simulink model "pospoli_XY_traiettoria_discretizzato"  (R2020b)
settings: Solver=VariableStepAuto  StartTime=0.0  StopTime=3  RelTol=1e-3
values from neighbouring files (symbols this model uses):
  Acc_asse_x = []    [main_Strategia_di_pilotaggio.m]
  Acc_asse_y = []    [main_Strategia_di_pilotaggio.m]
  Gppx_agg_rc = 0.4    [main_Strategia_di_pilotaggio.m]
  Gppx_agg_rm = 1    [main_Strategia_di_pilotaggio.m]
  Gppy_agg_rc = 0.8    [main_Strategia_di_pilotaggio.m]
  Gppy_agg_rm = 1    [main_Strategia_di_pilotaggio.m]
  mx = config_dc_x(parx)    [Main_traiettoria.m]    (also in Main_traiettoria_ordinato.m; main_Strategia_di_pilotaggio.m)
  my = config_dc_y(pary)    [Main_traiettoria.m]    (also in Main_traiettoria_ordinato.m; main_Strategia_di_pilotaggio.m)
  ppx_c = pos_poli_cc_x(mx, acx, 2)    [main_Strategia_di_pilotaggio.m]
  ppx_m = pos_poli_cc_x(mx, acx, 1)    [main_Strategia_di_pilotaggio.m]
  ppy_c = pos_poli_cc_y(my, acy, 2)    [main_Strategia_di_pilotaggio.m]
  ppy_m = pos_poli_cc_y(my, acy, 1)    [main_Strategia_di_pilotaggio.m]
  time = 0:tf/np:tf    [Main_traiettoria.m]    (also in Main_traiettoria_ordinato.m = 0:passo:tsim)
  Vel_asse_x = []    [main_Strategia_di_pilotaggio.m]
  Vel_asse_y = []    [main_Strategia_di_pilotaggio.m]
  x = zeros(length(time),1)    [Main_traiettoria.m]    (also in Main_traiettoria_ordinato.m; main_Strategia_di_pilotaggio.m = [])
  y = zeros(length(time),1)    [Main_traiettoria.m]    (also in Main_traiettoria_ordinato.m; main_Strategia_di_pilotaggio.m = [])
undefined symbols (not defined in the file or in its folder): accelerazioni, accelerazioniy, ci_x, ci_y, interpolazione_tempi, parx, pary
libraries: simulink x6
settings Model: Creator=stefa  LastModifiedBy=user
settings DebuggingCC: SFMachineParentedDataDiag=error

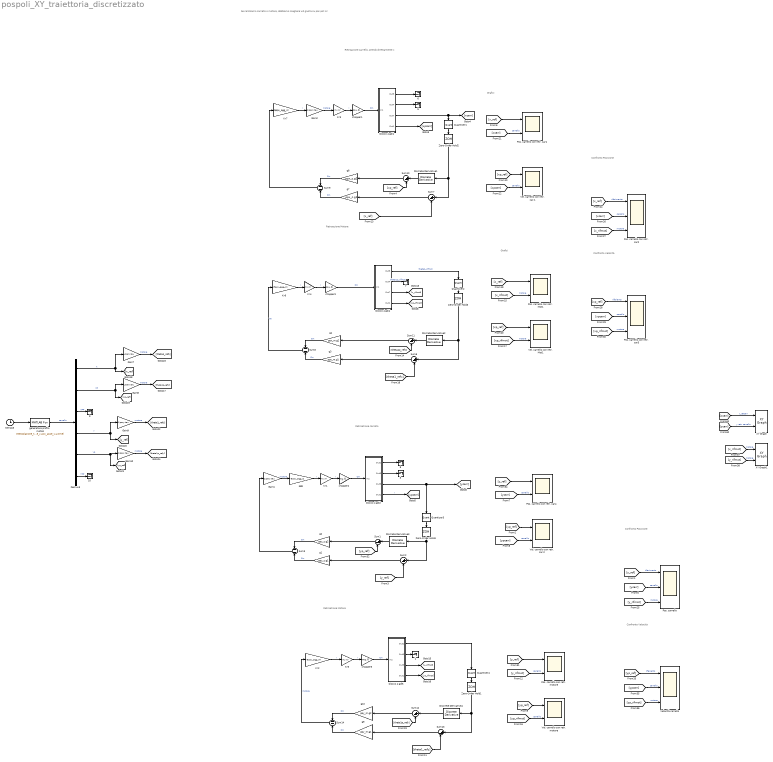
== system pospoli_XY_traiettoria_discretizzato ==
  note: Confronto Posizione
  note: Confronto
      | Velocità
  note: Retroazione Motore
  note: Grafici
  note: Grafici
  note: Retroazione carrello, prendo direttamente x
  note: Retroazione carrello
  note: Confronto
      | Velocità
  note: Retroazione Motore
  note: Confronto Posizione
  note: Se cambiamo carrello o motore, dobbiamo scegliere w0 giusta su pos poli cc
   {1,3,5..10} (8 alike) : Terminator
  Demux3 : Demux  Outputs=6
  Discrete Derivative1 : simulink/Discrete/Discrete Derivative  gainval=1  ICPrevScaledInput=0.0  OutMin=[]  OutMax=[]  OutDataType=fixdt(1, 16)  OutScaling=2^-10  DoSatur=off
  Discrete Derivative2 : simulink/Discrete/Discrete Derivative  gainval=1.0  ICPrevScaledInput=0.0  OutMin=[]  OutMax=[]  OutDataType=fixdt(1, 16)  OutScaling=2^-10  DoSatur=off
  Discrete Derivative3 : simulink/Discrete/Discrete Derivative  gainval=1  ICPrevScaledInput=0.0  OutMin=[]  OutMax=[]  OutDataType=fixdt(1, 16)  OutScaling=2^-10  DoSatur=off
  Discrete Derivative4 : simulink/Discrete/Discrete Derivative  gainval=1.0  ICPrevScaledInput=0.0  OutMin=[]  OutMax=[]  OutDataType=fixdt(1, 16)  OutScaling=2^-10  DoSatur=off
  Gain1 : Gain  Gain=1/pary.tau
  Gain10 : Gain  Gain=1/pary.tau
  Gain2 : Gain  Gain=1/parx.tau
  Gain7 : Gain  Gain=1/parx.tau
  Gain8 : Gain  Gain=1/parx.tau
  Gain9 : Gain  Gain=1/pary.tau
  Kr1 : Gain  Gain=my.Kr
  Kr2 : Gain  Gain=Gppy_agg_rm
  Kr3 : Gain  Gain=mx.Kr
  Kr4 : Gain  Gain=mx.Kr
  Kr5 : Gain  Gain=my.Kr
  Kr6 : Gain  Gain=Gppx_agg_rm
  Kr7 : Gain  Gain=Gppx_agg_rc
  "Pos. carrello " : Scope  NumInputPorts=3
  Pos. carrello con retr. Mot1 : Scope  NumInputPorts=2
  Pos. carrello con retr. car1 : Scope  NumInputPorts=2
  Pos. carrello con retr. car2 : Scope  NumInputPorts=3
  Pos. carrello con retr. car3 : Scope  NumInputPorts=3
  Pos. carrello con retr. car4 : Scope  NumInputPorts=2
  Pos. carrello con retr. motore : Scope  NumInputPorts=2
  Quantizer{1..4} (4 alike) : Quantizer  QuantizationInterval=10/4096
  Sum{1..2,6..7,10..13} (8 alike) : Sum  Inputs=|+-
  Sum{3,8..9,14} (4 alike) : Sum  Inputs=--
  Vel. carrello con retr. Mot1 : Scope  NumInputPorts=2
  Vel. carrello con retr. car.1 : Scope  NumInputPorts=2
  Vel. carrello con retr. car.2 : Scope  NumInputPorts=2
  Vel. carrello con retr. motore : Scope  NumInputPorts=2
  Velocità carrello : Scope  NumInputPorts=3
  XY Graph : simulink/Sinks/XY Graph  xmin=-0.5  xmax=0.5  ymin=-0.5  ymax=0.5  st=-1
  XY Graph1 : simulink/Sinks/XY Graph  xmin=-0.5  xmax=0.5  ymin=-0.5  ymax=0.5  st=-1
  Zero-Order Hold{1..4} (4 alike) : ZeroOrderHold  SampleTime=0.001
  agg : Gain  Gain=Gppy_agg_rc
  blocco 4 gdl1 : Subsystem
  blocco 4 gdl2 : Subsystem
  blocco 4 gdl4 : Subsystem
  blocco 4 gdl5 : Subsystem
  chopper1 : Gain  Gain=mx.K
  chopper2 : Gain  Gain=my.K
  chopper3 : Gain  Gain=mx.K
  chopper5 : Gain  Gain=my.K
  g1 : Gain  Gain=ppy_c.g1
  g10 : Gain  Gain=ppy_m.g2
  g2 : Gain  Gain=ppy_c.g2
  g3 : Gain  Gain=ppx_m.g1
  g4 : Gain  Gain=ppx_m.g2
  g7 : Gain  Gain=ppx_c.g1
  g8 : Gain  Gain=ppx_c.g2
  g9 : Gain  Gain=ppy_m.g1
  generatore profilo moto3 : MATLABFcn  MATLABFcn=interpolazione_tempi(x,Vel_asse_x,Acc_asse_x,y,Vel_asse_y,Acc_asse_y,u,time)  OutputDimensions=6
  tempo3 : Clock
      settings: Decimation=tsim
  wires:
  blocco 4 gdl4/2(Out4) -> " 7"/1  "theta1p_rifmot"
  chopper3/1 -> blocco 4 gdl4/1(In1)  "Cm"
  Discrete Derivative2/1 -> Sum11/1
  Quantizer2/1 -> Zero-Order Hold3/1
  [xcarr] -> Pos. carrello con retr. car2/2  "carrello"
  [xp_rifmot] -> Pos. carrello con retr. car3/3  "motore"
  blocco 4 gdl4/1(Out3) -> Quantizer2/1  "theta1_rifmot"
  [theta1_refx] -> Sum6/2
  [xp_rifmot] -> Vel. carrello con retr. Mot1/2  "motore"
  [xp_ref] -> Vel. carrello con retr. car.1/1
  g4/1 -> Sum8/1  "Cm"
  Kr4/1 -> chopper3/1  "I"
  blocco 4 gdl1/3(Out7) -> Quantizer1/1, [xcarr]
  blocco 4 gdl1/4(Out1) -> [xpcarr]
  blocco 4 gdl4/4(Out1) -> [xp_rifmot]
  [xp_ref] -> Sum10/2
  blocco 4 gdl4/3(Out7) -> [x_rifmot]
  g7/1 -> Sum9/2  "Cm"
  chopper1/1 -> blocco 4 gdl1/1(In1)  "Cm"
  [x_rifmot] -> Pos. carrello con retr. Mot1/2  "motore"
  g8/1 -> Sum9/1  "Cm"
  blocco 4 gdl1/1(Out3) -> " 6"/1
  [x_ref] -> Sum7/2
  [xpcarr] -> Pos. carrello con retr. car3/2  "carrello"
  Sum11/1 -> g4/1
  [x_ref] -> Pos. carrello con retr. car2/1  "riferimento"
  [xp_ref] -> Vel. carrello con retr. Mot1/1
  blocco 4 gdl1/2(Out4) -> " 5"/1
  [x_ref] -> Pos. carrello con retr. Mot1/1
  [xp_ref] -> Pos. carrello con retr. car3/1  "riferiento"
  [xpcarr] -> Vel. carrello con retr. car.1/2  "carrello"
  Quantizer1/1 -> Zero-Order Hold2/1
  Sum6/1 -> g3/1
  [xcarr] -> Pos. carrello con retr. car1/2  "carrello"
  Discrete Derivative1/1 -> Sum10/1
  [x_rifmot] -> Pos. carrello con retr. car2/3  "motore"
  [theta1p_refx] -> Sum11/2
  g3/1 -> Sum8/2  "Cm"
  Sum10/1 -> g8/1
  [x_ref] -> Pos. carrello con retr. car1/1
  Sum7/1 -> g7/1
  Kr3/1 -> chopper1/1  "I"
  [y_ref] -> Pos. carrello con retr. motore/1
  Sum12/1 -> g10/1
  blocco 4 gdl5/4(Out1) -> [yp_rifmot]
  blocco 4 gdl5/3(Out3) -> [y_rifmot]
  g2/1 -> Sum3/1  "Cm"
  chopper5/1 -> blocco 4 gdl5/1(In2)  "Cm"
  [ycarr] -> Pos. carrello con retr. car4/2  "carrello"
  blocco 4 gdl2/3(Out3) -> [ycarr], Quantizer3/1
  [yp_ref] -> Vel. carrello con retr. car.2/1
  Sum2/1 -> g1/1
  blocco 4 gdl2/4(Out1) -> [ypcarr]  "I"
  blocco 4 gdl5/2(Out5) -> " 1"/1
  [ypcarr] -> Velocità carrello/2  "carrello"
  chopper2/1 -> blocco 4 gdl2/1(In2)  "Cm"
  [y_ref] -> Pos. carrello con retr. car4/1
  Kr5/1 -> chopper5/1  "I"
  Sum13/1 -> g9/1
  [yp_ref] -> Vel. carrello con retr. motore/1
  Sum3/1 -> Gain1/1
  [theta1_refy] -> Sum13/2
  [y_ref] -> Sum2/2
  [ycarr] -> "Pos. carrello "/2  "carrello"
  Discrete Derivative4/1 -> Sum12/1
  g1/1 -> Sum3/2  "Cm"
  [y_rifmot] -> Pos. carrello con retr. motore/2  "carrello"
  g9/1 -> Sum14/2  "Cm"
  blocco 4 gdl2/1(Out2) -> " 8"/1
  Quantizer4/1 -> Zero-Order Hold1/1
  blocco 4 gdl2/2(Out5) -> " 3"/1
  [yp_rifmot] -> Velocità carrello/3  "motore"
  [theta1p_refy] -> Sum12/2
  [yp_ref] -> Velocità carrello/1  "riferiento"
  [yp_ref] -> Sum1/2
  blocco 4 gdl5/1(Out2) -> Quantizer4/1
  Sum1/1 -> g2/1
  [y_rifmot] -> "Pos. carrello "/3  "motore"
  Zero-Order Hold4/1 -> Discrete Derivative3/1, Sum2/1
  [yp_rifmot] -> Vel. carrello con retr. motore/2  "carrello"
  Zero-Order Hold1/1 -> Sum13/1, Discrete Derivative4/1
  Quantizer3/1 -> Zero-Order Hold4/1
  Discrete Derivative3/1 -> Sum1/1
  [y_ref] -> "Pos. carrello "/1  "riferimento"
  Kr1/1 -> chopper2/1  "I"
  [ypcarr] -> Vel. carrello con retr. car.2/2  "carrello"
  g10/1 -> Sum14/1  "Cm"
  Demux3/2 -> Gain8/1, [xp_ref]  "XP"
  Gain10/1 -> [theta1p_refy]  "motore"
  Demux3/4 -> [y_ref], Gain9/1  "Y"
  Demux3/1 -> [x_ref], Gain7/1  "X"
  Gain8/1 -> [theta1p_refx]  "motore"
  tempo3/1 -> generatore profilo moto3/1
  Demux3/6 -> " 10"/1  "YPP"
  Demux3/3 -> " 9"/1  "XPP"
  generatore profilo moto3/1 -> Demux3/1  "carrello"
  Demux3/5 -> [yp_ref], Gain10/1  "YP"
  Gain7/1 -> [theta1_refx]  "motore"
  Gain9/1 -> [theta1_refy]  "motore"
  [ycarr] -> XY Graph/2  "y retr. carrello"
  [xcarr] -> XY Graph/1  "x_retcarr"
  Zero-Order Hold2/1 -> Sum7/1, Discrete Derivative1/1
  Zero-Order Hold3/1 -> Discrete Derivative2/1, Sum6/1
  Gain2/1 -> Kr3/1  "motore"
  Gain1/1 -> agg/1  "motore"
  agg/1 -> Kr1/1  "I"
  [x_rifmot] -> XY Graph1/1  "motore"
  [y_rifmot] -> XY Graph1/2  "motore"
  Kr2/1 -> Kr5/1  "I"
  Sum14/1 -> Kr2/1  "motore"
  Kr6/1 -> Kr4/1  "I"
  Sum8/1 -> Kr6/1  "Va"
  Kr7/1 -> Gain2/1  "I"
  Sum9/1 -> Kr7/1

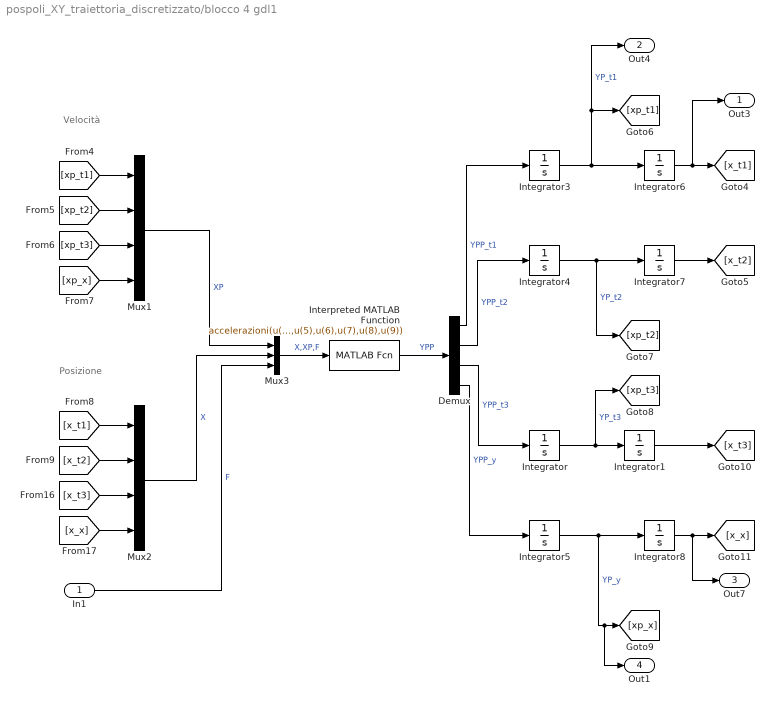
== system pospoli_XY_traiettoria_discretizzato/blocco 4 gdl1 ==
  note: Posizione
  note: Velocità
  In1 : Inport
  Demux : Demux
  Integrator{,3..5} (4 alike) : Integrator
  Integrator1 : Integrator  InitialCondition=ci_x(3)
  Integrator6 : Integrator  InitialCondition=ci_x(1)
  Integrator7 : Integrator  InitialCondition=ci_x(2)
  Integrator8 : Integrator  InitialCondition=ci_x(4)
  Interpreted MATLAB Function : MATLABFcn  MATLABFcn=accelerazioni(u(1),u(2),u(3),u(4),u(5),u(6),u(7),u(8),u(9))  OutputDimensions=4
  Mux1 : Mux
  Mux2 : Mux
  Mux3 : Mux  Inputs=3
  Out3 : Outport
  Out4 : Outport  Port=2
  Out7 : Outport  Port=3
  Out1 : Outport  Port=4
  wires:
  [xp_t3] -> Mux1/3
  Interpreted MATLAB Function/1 -> Demux/1  "YPP"
  Integrator3/1 -> Out4/1, [xp_t1], Integrator6/1  "YP_t1"
  Integrator8/1 -> Out7/1, [x_x]
  Integrator7/1 -> [x_t2]
  [xp_x] -> Mux1/4
  [x_t1] -> Mux2/1
  Mux1/1 -> Mux3/1  "XP"
  [x_x] -> Mux2/4
  Demux/3 -> Integrator/1  "YPP_t3"
  Integrator/1 -> Integrator1/1, [xp_t3]  "YP_t3"
  Mux2/1 -> Mux3/2  "X"
  Integrator6/1 -> Out3/1, [x_t1]
  Integrator5/1 -> Out1/1, [xp_x], Integrator8/1  "YP_y"
  [xp_t2] -> Mux1/2
  Mux3/1 -> Interpreted MATLAB Function/1  "X,XP,F"
  [x_t3] -> Mux2/3
  In1/1 -> Mux3/3  "F"
  Demux/4 -> Integrator5/1  "YPP_y"
  Integrator4/1 -> [xp_t2], Integrator7/1  "YP_t2"
  Integrator1/1 -> [x_t3]
  [xp_t1] -> Mux1/1
  [x_t2] -> Mux2/2
  Demux/2 -> Integrator4/1  "YPP_t2"
  Demux/1 -> Integrator3/1  "YPP_t1"

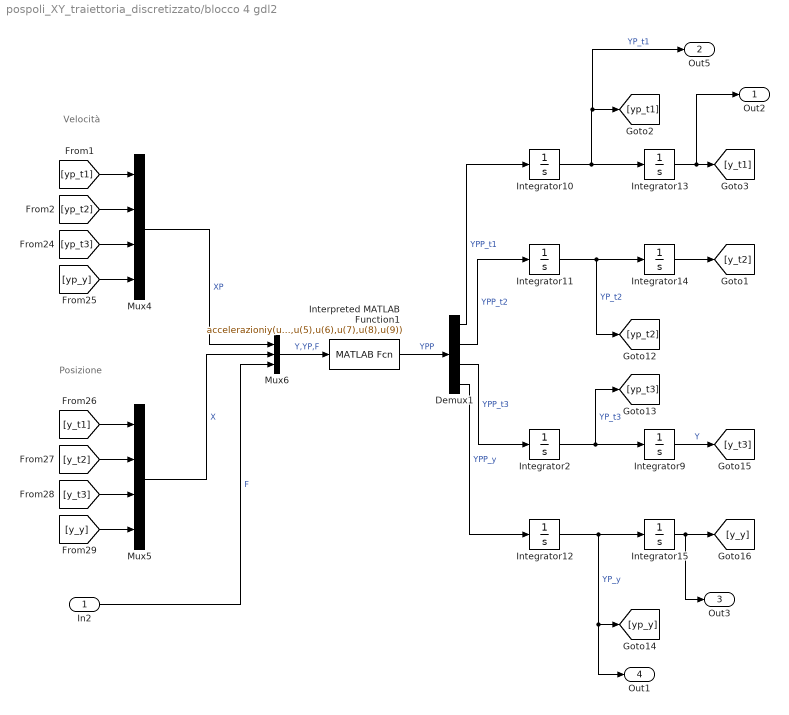
== system pospoli_XY_traiettoria_discretizzato/blocco 4 gdl2 ==
  note: Posizione
  note: Velocità
  In2 : Inport
  Demux1 : Demux
  Integrator{2,10..12} (4 alike) : Integrator
  Integrator13 : Integrator  InitialCondition=ci_y(1)
  Integrator14 : Integrator  InitialCondition=ci_y(2)
  Integrator15 : Integrator  InitialCondition=ci_y(4)
  Integrator9 : Integrator  InitialCondition=ci_y(3)
  Interpreted MATLAB Function1 : MATLABFcn  MATLABFcn=accelerazioniy(u(1),u(2),u(3),u(4),u(5),u(6),u(7),u(8),u(9))  OutputDimensions=4
  Mux4 : Mux
  Mux5 : Mux
  Mux6 : Mux  Inputs=3
  Out2 : Outport
  Out5 : Outport  Port=2
  Out3 : Outport  Port=3
  Out1 : Outport  Port=4
  wires:
  Integrator15/1 -> Out3/1, [y_y]
  [yp_t2] -> Mux4/2
  [y_y] -> Mux5/4
  Demux1/2 -> Integrator11/1  "YPP_t2"
  Demux1/1 -> Integrator10/1  "YPP_t1"
  Mux6/1 -> Interpreted MATLAB Function1/1  "Y,YP,F"
  Demux1/3 -> Integrator2/1  "YPP_t3"
  Integrator2/1 -> [yp_t3], Integrator9/1  "YP_t3"
  Mux5/1 -> Mux6/2  "X"
  [y_t2] -> Mux5/2
  [y_t3] -> Mux5/3
  [yp_y] -> Mux4/4
  Integrator11/1 -> [yp_t2], Integrator14/1  "YP_t2"
  Integrator14/1 -> [y_t2]
  [yp_t3] -> Mux4/3
  In2/1 -> Mux6/3  "F"
  Integrator10/1 -> Out5/1, [yp_t1], Integrator13/1  "YP_t1"
  Demux1/4 -> Integrator12/1  "YPP_y"
  Mux4/1 -> Mux6/1  "XP"
  [yp_t1] -> Mux4/1
  [y_t1] -> Mux5/1
  Integrator9/1 -> [y_t3]  "Y"
  Integrator12/1 -> Out1/1, [yp_y], Integrator15/1  "YP_y"
  Integrator13/1 -> Out2/1, [y_t1]
  Interpreted MATLAB Function1/1 -> Demux1/1  "YPP"

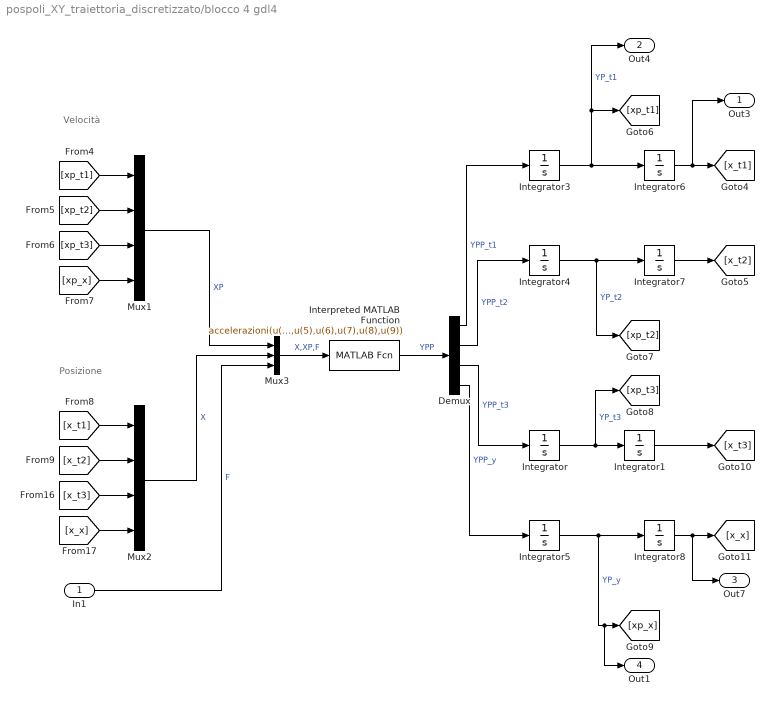
== system pospoli_XY_traiettoria_discretizzato/blocco 4 gdl4 ==
  note: Posizione
  note: Velocità
  In1 : Inport
  Demux : Demux
  Integrator{,3..5} (4 alike) : Integrator
  Integrator1 : Integrator  InitialCondition=ci_x(3)
  Integrator6 : Integrator  InitialCondition=ci_x(1)
  Integrator7 : Integrator  InitialCondition=ci_x(2)
  Integrator8 : Integrator  InitialCondition=ci_x(4)
  Interpreted MATLAB Function : MATLABFcn  MATLABFcn=accelerazioni(u(1),u(2),u(3),u(4),u(5),u(6),u(7),u(8),u(9))  OutputDimensions=4
  Mux1 : Mux
  Mux2 : Mux
  Mux3 : Mux  Inputs=3
  Out3 : Outport
  Out4 : Outport  Port=2
  Out7 : Outport  Port=3
  Out1 : Outport  Port=4
  wires:
  [xp_t3] -> Mux1/3
  Interpreted MATLAB Function/1 -> Demux/1  "YPP"
  Integrator3/1 -> Out4/1, [xp_t1], Integrator6/1  "YP_t1"
  Integrator8/1 -> Out7/1, [x_x]
  Integrator7/1 -> [x_t2]
  [xp_x] -> Mux1/4
  [x_t1] -> Mux2/1
  Mux1/1 -> Mux3/1  "XP"
  [x_x] -> Mux2/4
  Demux/3 -> Integrator/1  "YPP_t3"
  Integrator/1 -> Integrator1/1, [xp_t3]  "YP_t3"
  Mux2/1 -> Mux3/2  "X"
  Integrator6/1 -> Out3/1, [x_t1]
  Integrator5/1 -> Out1/1, [xp_x], Integrator8/1  "YP_y"
  [xp_t2] -> Mux1/2
  Mux3/1 -> Interpreted MATLAB Function/1  "X,XP,F"
  [x_t3] -> Mux2/3
  In1/1 -> Mux3/3  "F"
  Demux/4 -> Integrator5/1  "YPP_y"
  Integrator4/1 -> [xp_t2], Integrator7/1  "YP_t2"
  Integrator1/1 -> [x_t3]
  [xp_t1] -> Mux1/1
  [x_t2] -> Mux2/2
  Demux/2 -> Integrator4/1  "YPP_t2"
  Demux/1 -> Integrator3/1  "YPP_t1"

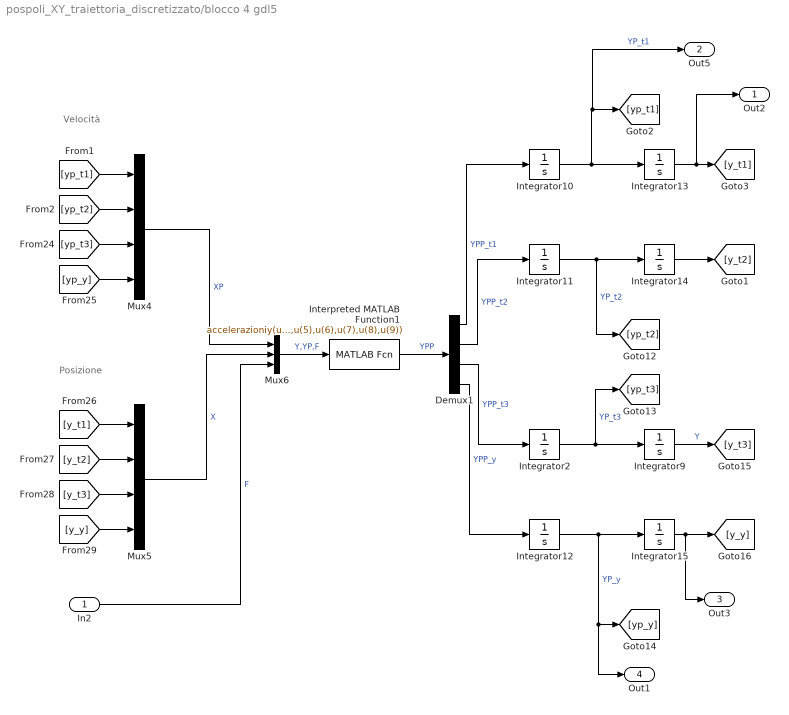
== system pospoli_XY_traiettoria_discretizzato/blocco 4 gdl5 ==
  note: Posizione
  note: Velocità
  In2 : Inport
  Demux1 : Demux
  Integrator{2,10..12} (4 alike) : Integrator
  Integrator13 : Integrator  InitialCondition=ci_y(1)
  Integrator14 : Integrator  InitialCondition=ci_y(2)
  Integrator15 : Integrator  InitialCondition=ci_y(4)
  Integrator9 : Integrator  InitialCondition=ci_y(3)
  Interpreted MATLAB Function1 : MATLABFcn  MATLABFcn=accelerazioniy(u(1),u(2),u(3),u(4),u(5),u(6),u(7),u(8),u(9))  OutputDimensions=4
  Mux4 : Mux
  Mux5 : Mux
  Mux6 : Mux  Inputs=3
  Out2 : Outport
  Out5 : Outport  Port=2
  Out3 : Outport  Port=3
  Out1 : Outport  Port=4
  wires:
  Mux4/1 -> Mux6/1  "XP"
  Integrator9/1 -> [y_t3]  "Y"
  [y_t2] -> Mux5/2
  [yp_t1] -> Mux4/1
  Integrator13/1 -> Out2/1, [y_t1]
  Demux1/4 -> Integrator12/1  "YPP_y"
  Integrator12/1 -> Out1/1, [yp_y], Integrator15/1  "YP_y"
  [yp_t3] -> Mux4/3
  Integrator2/1 -> [yp_t3], Integrator9/1  "YP_t3"
  Integrator11/1 -> [yp_t2], Integrator14/1  "YP_t2"
  Demux1/1 -> Integrator10/1  "YPP_t1"
  Integrator10/1 -> Out5/1, [yp_t1], Integrator13/1  "YP_t1"
  [y_t1] -> Mux5/1
  Mux5/1 -> Mux6/2  "X"
  [y_t3] -> Mux5/3
  Demux1/2 -> Integrator11/1  "YPP_t2"
  Interpreted MATLAB Function1/1 -> Demux1/1  "YPP"
  [yp_t2] -> Mux4/2
  [yp_y] -> Mux4/4
  Integrator14/1 -> [y_t2]
  Integrator15/1 -> Out3/1, [y_y]
  Demux1/3 -> Integrator2/1  "YPP_t3"
  Mux6/1 -> Interpreted MATLAB Function1/1  "Y,YP,F"
  [y_y] -> Mux5/4
  In2/1 -> Mux6/3  "F"
